simulink model "corrps_voltage"  (Simulink 7.8)
settings: Solver=ode45  StartTime=0.0  StopTime=10.0  RelTol=1e-3
values from neighbouring files (symbols this model uses):
  sofbctrl = param.sofbctrl    [simofb.m]
libraries: cstblocks x1
settings Model: Creator=danielot  LastModifiedBy=danielot
settings DebuggingCC: SolverPrmCheckMsg=none  ModelReferenceExtraNoncontSigs=none

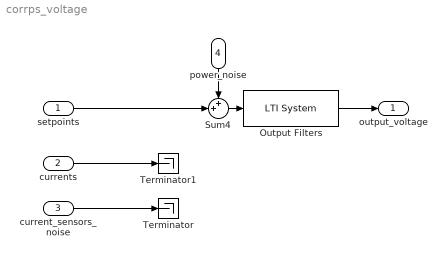
== system corrps_voltage ==
  setpoints : Inport  PortDimensions=ncorrsofb  SampleTime=sofbctrl.Ts
  currents : Inport  Port=2  PortDimensions=ncorrsofb
  current_sensors_noise : Inport  Port=3  PortDimensions=ncorrsofb
  power_noise : Inport  Port=4  PortDimensions=ncorrsofb
  Output Filters : cstblocks/LTI System  sys=corrpsfilter  IC=[]
  Sum4 : Sum  Inputs=++|  SampleTime=sofbctrl.Ts
  Terminator : Terminator
  Terminator1 : Terminator
  output_voltage : Outport
  wires:
  Output Filters/1 -> output_voltage/1
  Sum4/1 -> Output Filters/1
  setpoints/1 -> Sum4/2
  current_sensors_noise/1 -> Terminator/1
  currents/1 -> Terminator1/1
  power_noise/1 -> Sum4/1
